simulink model "Quadsim"  (R2012b)
settings: Solver=ode45  StartTime=0.0  StopTime=10.0  FixedStep=0.1  RelTol=1e-3
undefined symbols (not defined in the file): sigbuilder_block
settings Model: Creator=Estel  LastModifiedBy=Estel

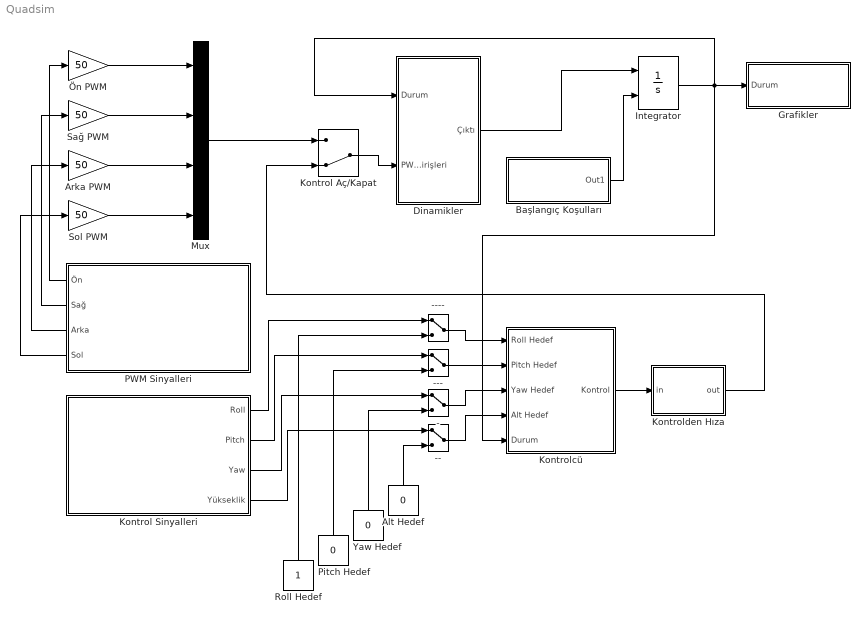
== system Quadsim ==
  - : ManualSwitch
  -- : ManualSwitch
  --- : ManualSwitch
  ---- : ManualSwitch
  Alt Hedef : Constant  Value=0
  Arka PWM : Gain  Gain=50
  Başlangıç Koşulları : Subsystem
  Dinamikler : Subsystem
  Grafikler : Subsystem
  Integrator : Integrator  InitialConditionSource=external
  Kontrol Aç/Kapat : ManualSwitch  CurrentSetting=0
  Kontrol Sinyalleri : Subsystem  Tag=STV Subsys  LoadFcn=sigbuilder_block('load');  StartFcn=sigbuilder_block('start');  StopFcn=sigbuilder_block('stop');  ClipboardFcn=sigbuilder_block('clipboard');  mask(Sigbuilder block){}
      mask help: Simulink:masks:SigbuilderBlock_MD
      mask init:
      | if ~strcmp(get_param(bdroot(gcbh),'SimulationStatus'),'stopped') tuvar = sigbuilder_block('maskInit'); end
      settings: CopyFcn=sigbuilder_block('copy');  DeleteFcn=sigbuilder_block('delete');  ModelCloseFcn=sigbuilder_block('modelClose');  PreSaveFcn=sigbuilder_block('preSave');  PauseFcn=sigbuilder_block('pause');  ContinueFcn=sigbuilder_block('continue');  NameChangeFcn=sigbuilder_block('namechange');  OpenFcn=sigbuilder_block('open',[6 31.5 1012.5 481.5 ]);  CloseFcn=sigbuilder_block('close');
      mask Display: plot(0, 0, 100, 100,[2, 2, 32, 32, 2], [68, 8, 8, 68, 68],[32, 2], [38, 38], [32, 19, 2],[53, 60, 44], [32, 17, 17, 2],[16, 16, 31, 31]);txt = getActiveGroup(gcbh);text(2, 100, txt,'verticalAlignment', 'top');
  Kontrolcü : Subsystem
  Kontrolden Hıza : MATLAB Function  TreatAsAtomicUnit=on
  Mux : Mux
  PWM Sinyalleri : Subsystem  Tag=STV Subsys  LoadFcn=sigbuilder_block('load');  StartFcn=sigbuilder_block('start');  StopFcn=sigbuilder_block('stop');  ClipboardFcn=sigbuilder_block('clipboard');  mask(Sigbuilder block){}
      mask help: Simulink:masks:SigbuilderBlock_MD
      mask init:
      | if ~strcmp(get_param(bdroot(gcbh),'SimulationStatus'),'stopped') tuvar = sigbuilder_block('maskInit'); end
      settings: CopyFcn=sigbuilder_block('copy');  DeleteFcn=sigbuilder_block('delete');  ModelCloseFcn=sigbuilder_block('modelClose');  PreSaveFcn=sigbuilder_block('preSave');  PauseFcn=sigbuilder_block('pause');  ContinueFcn=sigbuilder_block('continue');  NameChangeFcn=sigbuilder_block('namechange');  OpenFcn=sigbuilder_block('open',[6 28.5 1012.5 484.5 ]);  CloseFcn=sigbuilder_block('close');
      mask Display: plot(0, 0, 100, 100,[2, 2, 32, 32, 2], [68, 8, 8, 68, 68],[32, 2], [38, 38], [32, 19, 2],[53, 60, 44], [32, 17, 17, 2],[16, 16, 31, 31]);txt = getActiveGroup(gcbh);text(2, 100, txt,'verticalAlignment', 'top');
  Pitch Hedef : Constant  Value=0
  Roll Hedef : Constant
  Sağ PWM : Gain  Gain=50
  Sol PWM : Gain  Gain=50
  Yaw Hedef : Constant  Value=0
  Ön PWM : Gain  Gain=50
  wires:
  PWM Sinyalleri/4(Sol) -> Sol PWM/1
  PWM Sinyalleri/3(Arka) -> Arka PWM/1
  PWM Sinyalleri/2(Sağ) -> Sağ PWM/1
  PWM Sinyalleri/1(Ön) -> Ön PWM/1
  Arka PWM/1 -> Mux/3
  Sağ PWM/1 -> Mux/2
  Sol PWM/1 -> Mux/4
  Ön PWM/1 -> Mux/1
  Dinamikler/1(Çıktı) -> Integrator/1
  Integrator/1 -> Grafikler/1(Durum), Kontrolcü/5(Durum), Dinamikler/1(Durum)
  Başlangıç Koşulları/1(Out1) -> Integrator/2
  Mux/1 -> Kontrol Aç/Kapat/1
  Kontrol Aç/Kapat/1 -> Dinamikler/2(PWM Girişleri)
  Kontrolcü/1(Kontrol) -> Kontrolden Hıza/1(in)
  Kontrolden Hıza/1(out) -> Kontrol Aç/Kapat/2
  Kontrol Sinyalleri/1(Roll) -> ----/1
  Kontrol Sinyalleri/2(Pitch) -> ---/1
  Kontrol Sinyalleri/3(Yaw) -> -/1
  Kontrol Sinyalleri/4(Yükseklik) -> --/1
  Roll Hedef/1 -> ----/2
  Pitch Hedef/1 -> ---/2
  Yaw Hedef/1 -> -/2
  Alt Hedef/1 -> --/2
  --/1 -> Kontrolcü/4(Alt Hedef)
  -/1 -> Kontrolcü/3(Yaw Hedef)
  ---/1 -> Kontrolcü/2(Pitch Hedef)
  ----/1 -> Kontrolcü/1(Roll Hedef)

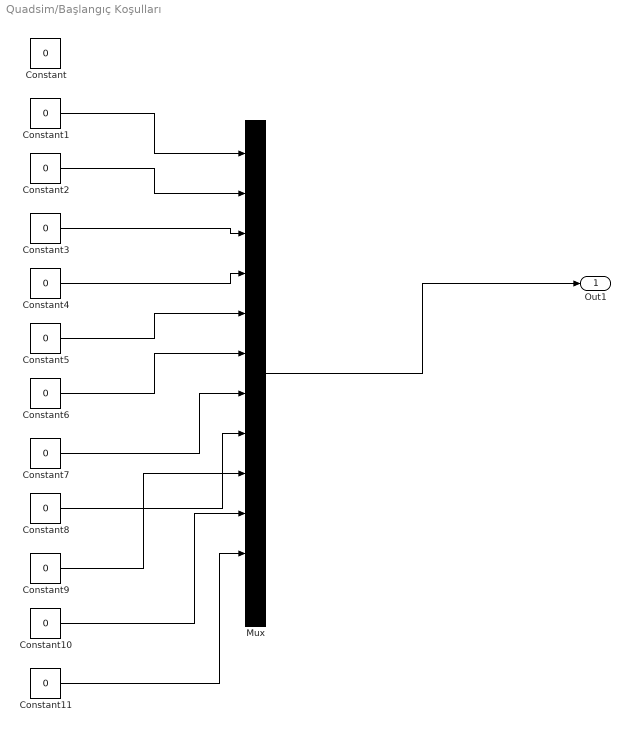
== system Quadsim/Başlangıç Koşulları ==
  Constant{,1..11} (12 alike) : Constant  Value=0
  Mux : Mux  Inputs=12
  Out1 : Outport
  wires:
  Constant3/1 -> Mux/3
  Constant4/1 -> Mux/4
  Constant5/1 -> Mux/5
  Constant2/1 -> Mux/2
  Constant6/1 -> Mux/6
  Constant1/1 -> Mux/1
  Constant7/1 -> Mux/7
  Constant8/1 -> Mux/8
  Constant9/1 -> Mux/9
  Constant10/1 -> Mux/10
  Constant11/1 -> Mux/11
  Mux/1 -> Out1/1

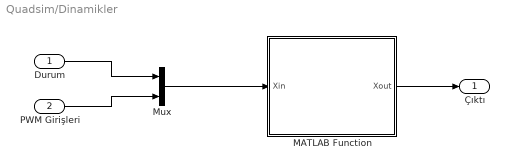
== system Quadsim/Dinamikler ==
  Durum : Inport
  PWM Girişleri : Inport  Port=2
  MATLAB Function : MATLAB Function  TreatAsAtomicUnit=on
  Mux : Mux  Inputs=2
  Çıktı : Outport
  wires:
  MATLAB Function/1(Xout) -> Çıktı/1
  PWM Girişleri/1 -> Mux/2
  Durum/1 -> Mux/1
  Mux/1 -> MATLAB Function/1(Xin)

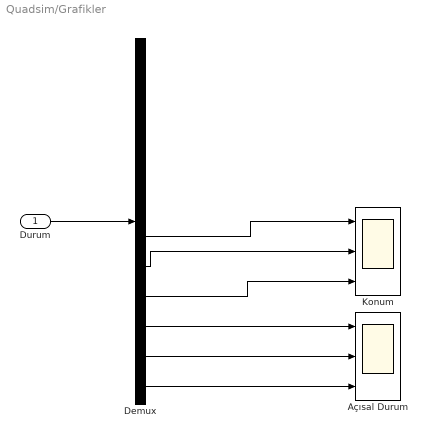
== system Quadsim/Grafikler ==
  Durum : Inport
  Açısal Durum : Scope  NumInputPorts=3
      settings: YMin=1790~-1~0.43  YMax=1920~1~0.455  MaxDataPoints=10000
  Demux : Demux  Outputs=12
  Konum : Scope  NumInputPorts=3
      settings: YMin=-5~-5~-5  YMax=5~5~5
  wires:
  Durum/1 -> Demux/1
  Demux/10 -> Açısal Durum/1
  Demux/11 -> Açısal Durum/2
  Demux/12 -> Açısal Durum/3
  Demux/7 -> Konum/1
  Demux/8 -> Konum/2
  Demux/9 -> Konum/3

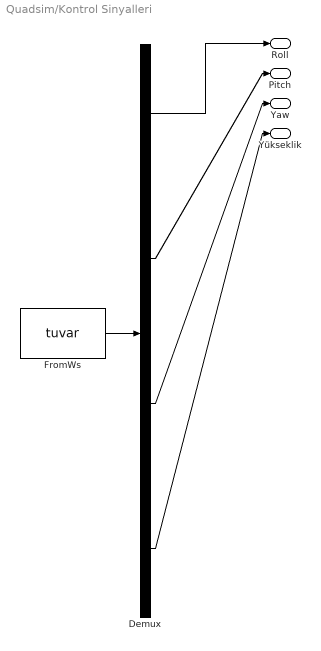
== system Quadsim/Kontrol Sinyalleri ==
  Demux : Demux  Tag=STV Demux
  FromWs : FromWorkspace  Tag=STV FromWs  VariableName=tuvar  SampleTime=0
      SigBuilderData=|
      | common.afterFinalStr = 'Extrapolate'
      | common.sampleTime = 0
      | dataSet.timeRange = [0 30]
      | dataSet.name = 'Group 1'
      | sbobj.Groups.Name = 'Group 1'
      | sbobj.Groups.Signals(1).Name = 'Roll'
      | sbobj.Groups.Signals(1).XData = [0 5 5 30]
      | sbobj.Groups.Signals(1).YData = [0 0 1 1]
      | sbobj.Groups.Signals(2).Name = 'Pitch'
      | sbobj.Groups.Signals(2).XData = [0 4 6 30]
      | sbobj.Groups.Signals(2).YData = [0 0 0 0]
      | sbobj.Groups.Signals(3).Name = 'Yaw'
      | sbobj.Groups.Signals(3).XData = [0 4 4 6 6 30]
      | sbobj.Groups.Signals(3).YData = [0 0 0 0 0 0]
      | sbobj.Groups.Signals(4).Name = 'Yükseklik'
      | sbobj.Groups.Signals(4).XData = [0 4 6 30]
      | sbobj.Groups.Signals(4).YData = [0 0 0 0]
      | sbobj.Groups.TimeRange = [0 30]
  Roll : Outport  Tag=STV Outport
  Pitch : Outport  Tag=STV Outport  Port=2
  Yaw : Outport  Tag=STV Outport  Port=3
  Yükseklik : Outport  Tag=STV Outport  Port=4
  wires:
  Demux/1 -> Roll/1
  FromWs/1 -> Demux/1
  Demux/2 -> Pitch/1
  Demux/3 -> Yaw/1
  Demux/4 -> Yükseklik/1

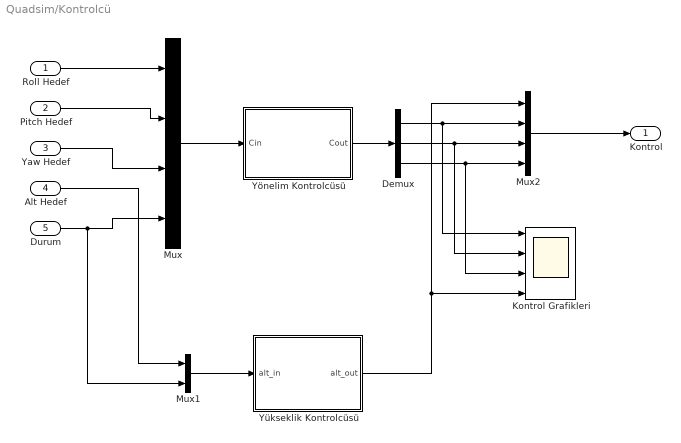
== system Quadsim/Kontrolcü ==
  Roll Hedef : Inport
  Pitch Hedef : Inport  Port=2
  Yaw Hedef : Inport  Port=3
  Alt Hedef : Inport  Port=4
  Durum : Inport  Port=5
  Demux : Demux  Outputs=3
  Kontrol Grafikleri : Scope  NumInputPorts=4
      settings: YMin=-1200~-1~-9~-10  YMax=100~1~0~120  SaveName=ScopeData2
  Mux : Mux
  Mux1 : Mux  Inputs=2
  Mux2 : Mux
  Yönelim Kontrolcüsü : MATLAB Function  TreatAsAtomicUnit=on
  Yükseklik Kontrolcüsü : MATLAB Function  TreatAsAtomicUnit=on
  Kontrol : Outport
  wires:
  Roll Hedef/1 -> Mux/1
  Pitch Hedef/1 -> Mux/2
  Yaw Hedef/1 -> Mux/3
  Durum/1 -> Mux1/2, Mux/4
  Mux/1 -> Yönelim Kontrolcüsü/1(Cin)
  Mux1/1 -> Yükseklik Kontrolcüsü/1(alt_in)
  Alt Hedef/1 -> Mux1/1
  Yönelim Kontrolcüsü/1(Cout) -> Demux/1
  Demux/1 -> Kontrol Grafikleri/1, Mux2/2
  Demux/2 -> Kontrol Grafikleri/2, Mux2/3
  Demux/3 -> Kontrol Grafikleri/3, Mux2/4
  Yükseklik Kontrolcüsü/1(alt_out) -> Kontrol Grafikleri/4, Mux2/1
  Mux2/1 -> Kontrol/1

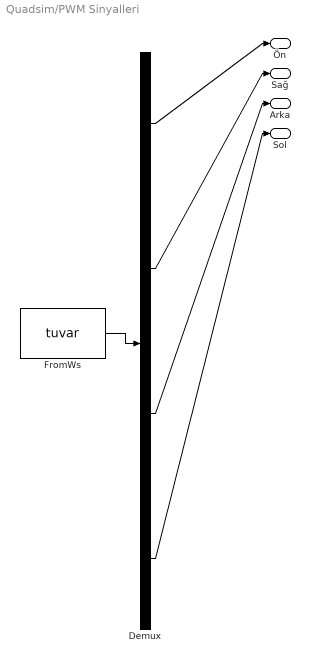
== system Quadsim/PWM Sinyalleri ==
  Demux : Demux  Tag=STV Demux
  FromWs : FromWorkspace  Tag=STV FromWs  VariableName=tuvar  SampleTime=0
      SigBuilderData=|
      | common.afterFinalStr = 'Extrapolate'
      | common.sampleTime = 0
      | dataSet.timeRange = [0 30]
      | dataSet.name = 'Group 1'
      | sbobj.Groups.Name = 'Group 1'
      | sbobj.Groups.Signals(1).Name = 'Ön'
      | sbobj.Groups.Signals(1).XData = [0 5 5 6 6 7 30]
      | sbobj.Groups.Signals(1).YData = [0.6 0.6 0.65 0.65 0.6 0.6 0.6]
      | sbobj.Groups.Signals(2).Name = 'Sağ'
      | sbobj.Groups.Signals(2).XData = [0 5 30]
      | sbobj.Groups.Signals(2).YData = [0.6 0.6 0.6]
      | sbobj.Groups.Signals(3).Name = 'Arka'
      | sbobj.Groups.Signals(3).XData = [0 5 5 6 6 7 30]
      | sbobj.Groups.Signals(3).YData = [0.6 0.6 0.55 0.55 0.6 0.6 0.6]
      | sbobj.Groups.Signals(4).Name = 'Sol'
      | sbobj.Groups.Signals(4).XData = [0 5 30]
      | sbobj.Groups.Signals(4).YData = [0.6 0.6 0.6]
      | sbobj.Groups.TimeRange = [0 30]
  Ön : Outport  Tag=STV Outport
  Sağ : Outport  Tag=STV Outport  Port=2
  Arka : Outport  Tag=STV Outport  Port=3
  Sol : Outport  Tag=STV Outport  Port=4
  wires:
  FromWs/1 -> Demux/1
  Demux/1 -> Ön/1
  Demux/2 -> Sağ/1
  Demux/3 -> Arka/1
  Demux/4 -> Sol/1

== matlab function Quadsim/Kontrolcü/Yönelim Kontrolcüsü ==
  data: Cin input; Cout output
function Cout  = yonelimKontrol(Cin)

global roll_i_error;

roll_set = Cin(1);
pitch_set = Cin(2);
yaw_set = Cin(3);
% x_dot = Cin(4);
% y_dot = Cin(5);
% z_dot = Cin(6);
roll_dot = Cin(7);
pitch_dot = Cin(8);
yaw_dot = Cin(9);
% x = Cin(10);
% y = Cin(11);
% z = Cin(12);
roll = Cin(13);
pitch = Cin(14);
yaw = Cin(15);

% PID DEĞERLERİ
roll_p = 1;
roll_i = 0;
roll_d = 0;

pitch_p = 0.5;
pitch_i = 0;
pitch_d = 0.175;

yaw_p = 5;
yaw_i = 0;
yaw_d = 10;

% KONTROL
roll_error = roll_set - roll;
pitch_error = pitch_set - pitch;
yaw_error = yaw_set - yaw;

roll_d_error = roll_dot;
pitch_d_error = pitch_dot;
yaw_d_error = yaw_dot;

%roll_i_error = roll_i_error + (roll_error*0.02);
%pitch_i_error = pitch_i_error + (pitch_error);
%yaw_i_error = yaw_i_error + (yaw_error*0.02);

roll_return = (roll_p*roll_error)-(roll_d*roll_d_error);
pitch_return = (pitch_p*pitch_error)-(pitch_d*pitch_d_error);
yaw_return = (yaw_p*yaw_error)-(yaw_d*yaw_d_error);

% pitch_return = (pitch_p*pitch_error)+(pitch_i*pitch_i_error)+(pitch_d*pitch_d_error)
% yaw_return = (yaw_p*yaw_error)+(yaw_i*yaw_i_error)+(yaw_d*yaw_d_error);

Cout = [0 0 0];
Cout(1) = roll_return;
Cout(2) = pitch_return;
Cout(3) = yaw_return;

end

== matlab function Quadsim/Dinamikler/MATLAB Function ==
  data: Xout output; Xin input
function Xout   = quadrosim(Xin)

arm_l = 0.23;
craft_m = 0.65;
Ixx = 7.5*10^(-3);
Iyy = 7.5*10^(-3);
Izz = 1.3*10^(-2);
b = 3.13*10^(-5);  % Thrust factor
d = 7.5*10^(-7);  % Drag factor
g = 9.81;

% DURUM DEĞİŞKENLERİ
X_dot = Xin(1);
Y_dot = Xin(2);
Z_dot = Xin(3);
Roll_dot = Xin(4);
Pitch_dot = Xin(5);
Yaw_dot = Xin(6);
X = Xin(7);
Y = Xin(8);
Z = Xin(9);
Roll = Xin(10);
Pitch = Xin(11);
Yaw = Xin(12);
% X_dot1 = X_dot;
% Y_dot1 = Y_dot;
% Z_dot1 = Z_dot;
% Roll_dot1 = Roll_dot;
% Pitch_dot1 = Pitch_dot;
% Yaw_dot1 = Yaw_dot;

% % GİRDİLER
F = Xin(13);
R = Xin(14);
B = Xin(15);
L = Xin(16);

% İTKİ HESAPLARI
TF = b*F^2;
TR = b*R^2;
TB = b*B^2;
TL = b*L^2;
D = d*(-F+R-B+L);

% SİSTEM DİNAMİĞİ
% Model
% X_ddot = -(1/craft_m) * (cos(Roll)*sin(Pitch)*cos(Yaw) + sin(Roll)*sin(Yaw))*(TF+TR+TB+TL);
% Y_ddot = -(1/craft_m) * (cos(Roll)*sin(Pitch)*sin(Yaw) + sin(Roll)*cos(Yaw))*(TF+TR+TB+TL);
% z_craft_component = (1/craft_m)*cos(Roll)*cos(Pitch)*(TF+TR+TB+TL);
% Z_ddot = g - z_craft_component;
% Roll_ddot = Pitch_dot*Yaw_dot*(Iyy-Izz)/Ixx + ((arm_l)/Ixx)*(-TR+TL);
% Pitch_ddot = Roll_dot*Yaw_dot*(Izz-Ixx)/Iyy + ((arm_l)/Iyy)*(TF-TB);
% Yaw_ddot = Roll_dot*Pitch_dot*(Ixx-Iyy)/Izz + (D)/Izz;

% Basitleştirilmiş (Lineerize edilmiş) model
X_ddot = -(1/craft_m) * (cos(Roll)*sin(Pitch)*cos(Yaw) + sin(Roll)*sin(Yaw))*(TF+TR+TB+TL);
Y_ddot = -(1/craft_m) * (cos(Roll)*sin(Pitch)*sin(Yaw) + sin(Roll)*cos(Yaw))*(TF+TR+TB+TL);
z_craft_component = (1/craft_m)*cos(Roll)*cos(Pitch)*(TF+TR+TB+TL);
Z_ddot = -g + z_craft_component;
Roll_ddot = ((arm_l)/Ixx)*(-TR+TL);
Pitch_ddot = ((arm_l)/Iyy)*(TF-TB);
Yaw_ddot = (D)/Izz;

% ÇIKTI
Xout = [X_ddot Y_ddot Z_ddot Roll_ddot Pitch_ddot Yaw_ddot X_dot Y_dot Z_dot Roll_dot Pitch_dot Yaw_dot];

end

== matlab function Quadsim/Kontrolcü/Yükseklik Kontrolcüsü ==
  data: alt_in input; alt_out output
function alt_out = yukseklikKontrol(alt_in)
%#codegen

altitude_set = alt_in(1);
% x_dot = alt_in(2);
% y_dot = alt_in(3);
z_dot = alt_in(4);
% roll_dot = alt_in(5);
% pitch_dot = alt_in(6);
% yaw_dot = alt_in(7);
% x = alt_in(8);
% y = alt_in(9);
z = alt_in(10);
% roll = alt_in(11);
% pitch = alt_in(12);
% yaw = alt_in(13);
% altitude_i_error = alt_in(14);
% altitude_last_pos = alt_in(15);

% PID DEĞERLERİ
altitude_p = 3;
altitude_i = 0;
altitude_d = 0.2;

% KONTROL
altitude_error = altitude_set - z;
%altitude_i_error = altitude_i_error + (altitude_error*0.02);
altitude_d_error = z_dot;
altitude_return = (altitude_p*altitude_error)-(altitude_d*altitude_d_error);
altitude_last_out = z;

alt_out = altitude_return;

end

== matlab function Quadsim/Kontrolden Hıza ==
  data: in input; out output
function out = c2s(in)
%#codegen
arm_l = 0.23;
craft_m = 0.65;
b = 3.13*10^(-5);  % Thrust factor
d = 7.5*10^(-7);  % Drag factor
g = 9.81;

U = [0 0 0 0];
U(1) = craft_m*g;
%U(1) = in(1);
U(2) = in(2);
U(3) = in(3);
U(4) = in(4);

MM = [  1/(4*b)     0               1/(2*arm_l*b)   -1/(4*d);
        1/(4*b)     -1/(2*arm_l*b)  0               1/(4*d);
        1/(4*b)     0               -1/(2*arm_l*b)  -1/(4*d);
        1/(4*b)     1/(2*arm_l*b)   0               1/(4*d)     ];
MA = MM * U';

Omd = sqrt(abs(MA));

out = [0 0 0 0];
out(1) = Omd(1);
out(2) = Omd(2);
out(3) = Omd(3);
out(4) = Omd(4);

end
